simulink model "Model_silnika_PID_ulamkowy"  (R2024a)
settings: Solver=ode23  StartTime=0.0  StopTime=czas_symulacji  MinStep=1e-5  RelTol=1e-2
undefined symbols (not defined in the file or in its folder): Kd, Ki, Kp
libraries: fod x2, SignalEditorBlockLib x1
settings Model: Creator=kkucm  LastModifiedBy=krzysiek89
settings SolverCC: MaxConsecutiveMinStep=20  ZeroCrossAlgorithm=Adaptive  EnableFixedStepZeroCrossing=on  MaxZcBracketingIterations=1000
settings DebuggingCC: IgnoredZcDiagnostic=none
settings RTWCC: GPUComputeCapability=3.5

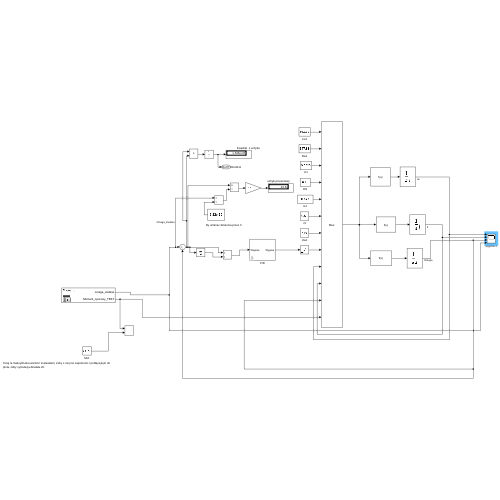
[thumbnail: Simulink's stored preview of the top-level diagram]
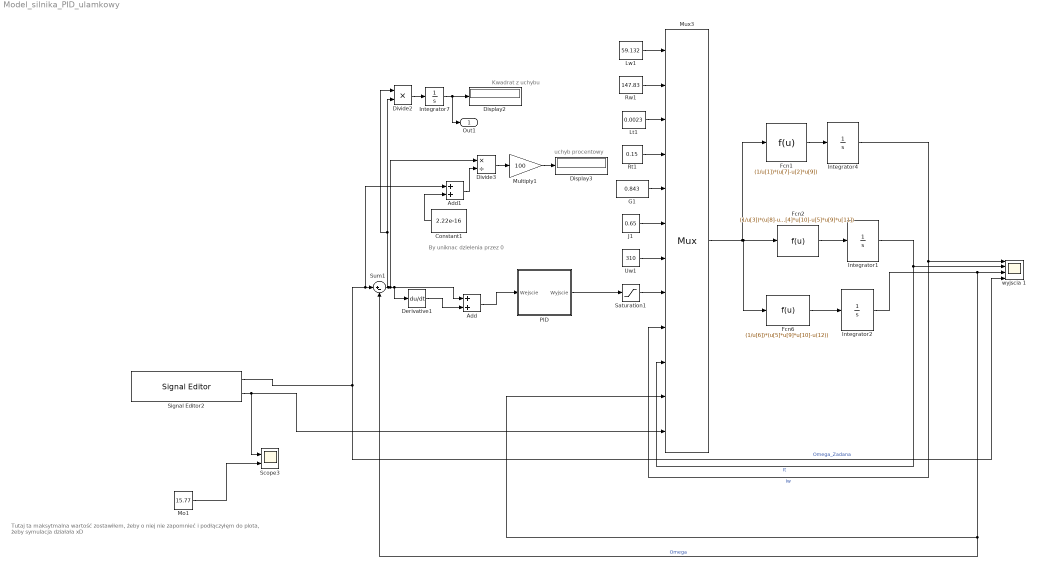
== system Model_silnika_PID_ulamkowy ==
  note: Kwadrat z uchybu
  note: Tutaj ta maksytmalna wartość zostawiłem, żeby o niej nie zapomnieć i podłączyłęm do plota, żeby symulacja działała xD
  note: uchyb procentowy
  note: By uniknac dzielenia przez 0
  Add : Sum
  Add1 : Sum
  Constant1 : Constant  Value=2.22e-16
  Derivative1 : Derivative
  Display2 : Display
  Display3 : Display
  Divide2 : Product  Inputs=**
  Divide3 : Product  Inputs=*/
  Fcn1 : Fcn  Expr=(1/u[1])*(u[7]-u[2]*u[9])
  Fcn2 : Fcn  Expr=(1/u[3])*(u[8]-u[4]*u[10]-u[5]*u[9]*u[11])
  Fcn6 : Fcn  Expr=(1/u[6])*(u[5]*u[9]*u[10]-u(12))
  G1 : Constant  Value=0.843  VectorParams1D=off
  Integrator1 : Integrator  InitialCondition=0.000001  LimitOutput=on  UpperSaturationLimit=1e4  LowerSaturationLimit=-1e4
  Integrator2 : Integrator  InitialCondition=0.000001  LimitOutput=on  UpperSaturationLimit=1e4  LowerSaturationLimit=-1e4
  Integrator4 : Integrator  InitialCondition=0.000001  LimitOutput=on  UpperSaturationLimit=1e4  LowerSaturationLimit=-1e4
  Integrator7 : Integrator  LowerSaturationLimit=1e-5
  J1 : Constant  Value=0.65
  Lt1 : Constant  Value=0.0023
  Lw1 : Constant  Value=59.132
  Mo1 : Constant  Value=15.77
  Multiply1 : Gain  Gain=100
  Mux3 : Mux  Inputs=12
  PID : Subsystem  mask{P=Kp, I=Ki, D=Kd}
  Rt1 : Constant  Value=0.15
  Rw1 : Constant  Value=147.83
  Saturation1 : Saturate  UpperLimit=528  LowerLimit=0
  Scope3 : Scope  NumInputPorts=2
  Signal Editor2 : SignalEditorBlockLib/Signal Editor  FileName=omega_zadana.mat  ActiveScenario=Scenario  ActiveSignal=omaga_zadana  IsBus=off  OutputBusObjectStr=Bus: BusObject  SampleTime=0  ZeroCross=off  OutputAfterFinalValue=Setting to zero  Unit=inherit  PreserveSignalName=on  ApplySigPropsToAllScenarios=on  ApplySigPropsToAllSignals=off
  Sum1 : Sum  Inputs=|+-
  Uw1 : Constant  Value=310
  wyjscia 1 : Scope  NumInputPorts=4
  Out1 : Outport  SignalName=Out1111
  wires:
  Saturation1/1 -> Mux3/8
  Constant1/1 -> Add1/2
  Rw1/1 -> Mux3/2
  Mux3/1 -> Fcn1/1, Fcn6/1, Fcn2/1
  Uw1/1 -> Mux3/7
  J1/1 -> Mux3/6
  Signal Editor2/2 -> Mux3/12, Scope3/1
  Signal Editor2/1 -> wyjscia 1/4, Add1/1, Sum1/1  "Omega_Zadana"
  Divide2/1 -> Integrator7/1
  Integrator7/1 -> Out1/1, Display2/1
  Sum1/1 -> Divide2/1, Divide2/2, Divide3/1, Derivative1/1, Add/1
  Fcn2/1 -> Integrator1/1
  Fcn1/1 -> Integrator4/1
  Mo1/1 -> Scope3/2
  Integrator2/1 -> Mux3/11, Sum1/2, wyjscia 1/3  "Omega"
  Lt1/1 -> Mux3/3
  Divide3/1 -> Multiply1/1
  Multiply1/1 -> Display3/1
  G1/1 -> Mux3/5
  Fcn6/1 -> Integrator2/1
  Add1/1 -> Divide3/2
  Integrator1/1 -> Mux3/10, wyjscia 1/2  "It"
  Rt1/1 -> Mux3/4
  Integrator4/1 -> Mux3/9, wyjscia 1/1  "Iw"
  Lw1/1 -> Mux3/1
  PID/1(Wyjscie) -> Saturation1/1
  Derivative1/1 -> Add/2
  Add/1 -> PID/1(Wejscie)

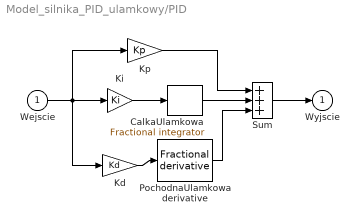
== system Model_silnika_PID_ulamkowy/PID ==
  Wejscie : Inport
  "CalkaUlamkowa " : fod/Fractional integrator  gam=Alfa  ww=[0.01; 100]  n=9  nFod=off
      settings: SourceProductName=FOMCON Toolbox
  Kd : Gain  Gain=Kd  SaturateOnIntegerOverflow=on  OutDataTypeStr=Inherit: Same as input  ParamDataTypeStr=Inherit: Same as input
  Ki : Gain  Gain=Ki  SaturateOnIntegerOverflow=on  OutDataTypeStr=Inherit: Same as input  ParamDataTypeStr=Inherit: Same as input
  Kp : Gain  Gain=Kp  SaturateOnIntegerOverflow=on  OutDataTypeStr=Inherit: Same as input  ParamDataTypeStr=Inherit: Same as input
  PochodnaUlamkowa derivative : fod/Fractional derivative  gam=Beta  ww=[0.01; 100]  n=9  nFod=off
      settings: SourceProductName=FOMCON Toolbox
  Sum : Sum  Inputs=+++  InputSameDT=on  SaturateOnIntegerOverflow=on  OutDataTypeStr=Inherit: Same as first input
  Wyjscie : Outport  InitialOutput=0
  wires:
  Kd/1 -> PochodnaUlamkowa derivative/1
  Wejscie/1 -> Kp/1, Ki/1, Kd/1
  Sum/1 -> Wyjscie/1
  PochodnaUlamkowa derivative/1 -> Sum/3
  "CalkaUlamkowa "/1 -> Sum/2
  Kp/1 -> Sum/1
  Ki/1 -> "CalkaUlamkowa "/1
